simulink subsystem "Stabilized"  (R2024a)
settings: Solver=VariableStepAuto  StartTime=0.0  StopTime=10.0  RelTol=1e-3
undefined symbols (not defined in the file): vehicle
settings Model: Creator=gurt1  LastModifiedBy=gurt1

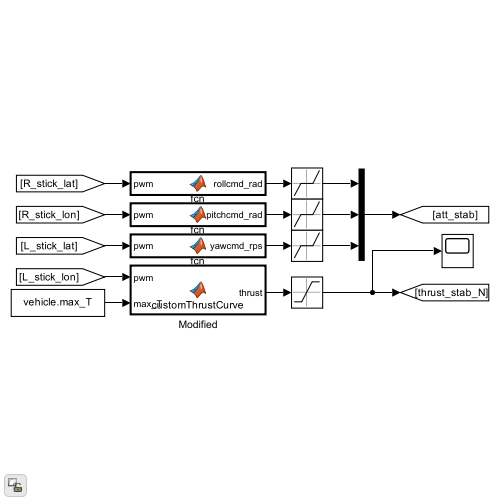
[thumbnail: Simulink's stored preview of the top-level diagram]
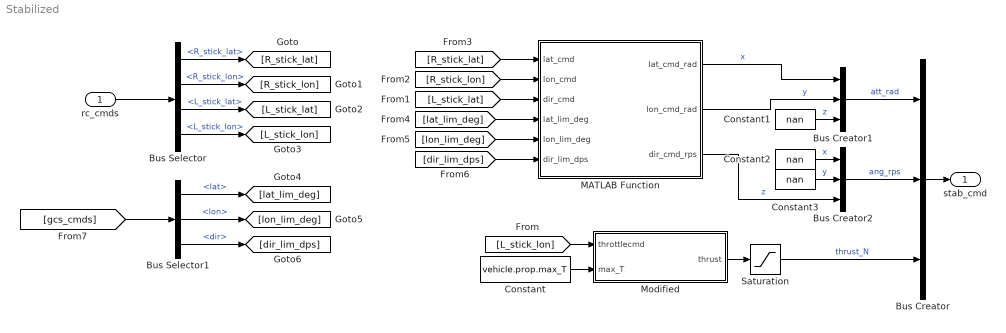
== system Stabilized ==
  rc_cmds : Inport
  Bus Creator : BusCreator  Inputs=3
  Bus Creator1 : BusCreator  Inputs=3
  Bus Creator2 : BusCreator  Inputs=3
  Bus Selector : BusSelector  OutputSignals=sticks.R_stick_lat,sticks.R_stick_lon,sticks.L_stick_lat,sticks.L_stick_lon
  Bus Selector1 : BusSelector  OutputSignals=OL.stabilized.lim.lat,OL.stabilized.lim.lon,OL.stabilized.lim.dir
  Constant : Constant  Value=vehicle.prop.max_T
  Constant1 : Constant  Value=nan
  Constant2 : Constant  Value=nan
  Constant3 : Constant  Value=nan
  MATLAB Function : MATLAB Function  TreatAsAtomicUnit=on
  Modified : MATLAB Function  TreatAsAtomicUnit=on
  Saturation : Saturate  UpperLimit=100  LowerLimit=0
  stab_cmd : Outport
  wires:
  [R_stick_lat] -> MATLAB Function/1(lat_cmd)
  Constant/1 -> Modified/2(max_T)
  [L_stick_lat] -> MATLAB Function/3(dir_cmd)
  [R_stick_lon] -> MATLAB Function/2(lon_cmd)
  Modified/1(thrust) -> Saturation/1
  [L_stick_lon] -> Modified/1(throttlecmd)
  Saturation/1 -> Bus Creator/3  "thrust_N"
  Bus Selector/2 -> [R_stick_lon]  "<R_stick_lon>"
  Bus Selector/4 -> [L_stick_lon]  "<L_stick_lon>"
  Bus Selector/1 -> [R_stick_lat]  "<R_stick_lat>"
  Bus Selector/3 -> [L_stick_lat]  "<L_stick_lat>"
  rc_cmds/1 -> Bus Selector/1
  [gcs_cmds] -> Bus Selector1/1
  Bus Selector1/1 -> [lat_lim_deg]  "<lat>"
  Bus Selector1/2 -> [lon_lim_deg]  "<lon>"
  Bus Selector1/3 -> [dir_lim_dps]  "<dir>"
  [lat_lim_deg] -> MATLAB Function/4(lat_lim_deg)
  [lon_lim_deg] -> MATLAB Function/5(lon_lim_deg)
  [dir_lim_dps] -> MATLAB Function/6(dir_lim_dps)
  Bus Creator/1 -> stab_cmd/1
  Bus Creator1/1 -> Bus Creator/1  "att_rad"
  Bus Creator2/1 -> Bus Creator/2  "ang_rps"
  MATLAB Function/1(lat_cmd_rad) -> Bus Creator1/1  "x"
  MATLAB Function/2(lon_cmd_rad) -> Bus Creator1/2  "y"
  Constant1/1 -> Bus Creator1/3  "z"
  Constant2/1 -> Bus Creator2/1  "x"
  Constant3/1 -> Bus Creator2/2  "y"
  MATLAB Function/3(dir_cmd_rps) -> Bus Creator2/3  "z"

== matlab function Stabilized/MATLAB Function ==
  data: lat_cmd input; lat_cmd_rad output; lon_cmd input; dir_cmd input; lat_lim_deg input; lon_lim_deg input; dir_lim_dps input; lon_cmd_rad output; dir_cmd_rps output
function [lat_cmd_rad, lon_cmd_rad, dir_cmd_rps] = scaleCommands(lat_cmd, lon_cmd, dir_cmd, lat_lim_deg, lon_lim_deg, dir_lim_dps)

    % Scale roll command
    lat_cmd_rad = (lat_cmd * lat_lim_deg)*(pi/180);

    % Scale pitch command
    lon_cmd_rad = (lon_cmd * lon_lim_deg)*(pi/180);

    % Scale yaw command
    dir_cmd_rps = (dir_cmd * dir_lim_dps)*(pi/180);

end

== matlab function Stabilized/Modified ==
  data: throttlecmd input; thrust output; max_T input
function thrust = customThrustCurve(throttlecmd, max_T)

% Input throttlecmd is now in the range -1 to 1

% Normalize the input throttlecmd to a range of 0 to 100%
throttlecmd = ((throttlecmd + 1) / 2) * 100;

% Adjust max_T for 10% thrust fudge factor
max_T = max_T * 1.10;

% Custom equation for the range 34% to 64%
if throttlecmd >= 34 && throttlecmd <= 64
    thrust = ((((4.0474698070e-3)*throttlecmd^3) - (5.9809705749e-1*throttlecmd^2) + (2.9501350778e1*throttlecmd) - 4.3543415069e2)/100) * max_T;
elseif throttlecmd < 34
    % Linear mapping from 0 to 33% throttle command to 5% to 33% thrust command
    thrust = ((throttlecmd / 33) * 0.33) * max_T;
else
    % Linear mapping from 65% to 100% throttle command to 65% to 100% thrust command
    thrust = ((65 + 35 * ((throttlecmd - 64) / 36)) / 100) * max_T;
end

end
